simulink model "J52"  (R2015b)
settings: Solver=VariableStepAuto  StartTime=-10  StopTime=10.0  RelTol=1e-3
libraries: simulink x1
settings Model: Creator=Pouya  LastModifiedBy=Pouya

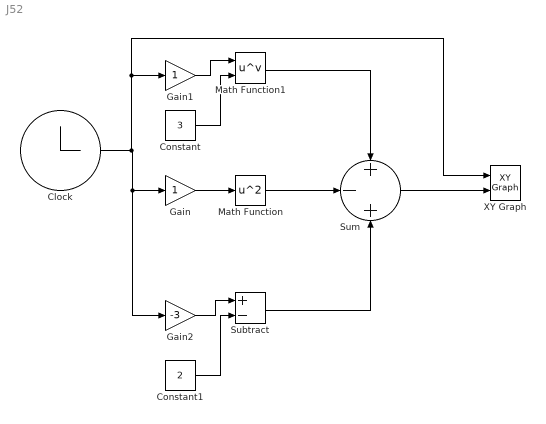
== system J52 ==
  Clock : Clock
  Constant : Constant  Value=3
  Constant1 : Constant  Value=2
  Gain : Gain
  Gain1 : Gain
  Gain2 : Gain  Gain=-3
  Math Function : Math  Operator=square  SaturateOnIntegerOverflow=on
  Math Function1 : Math  Operator=pow  SaturateOnIntegerOverflow=on
  Subtract : Sum  Inputs=+-
  Sum : Sum  Inputs=+-+
  XY Graph : simulink/Sinks/XY Graph  xmin=-4  xmax=4  ymin=-100  ymax=100  st=-1
  wires:
  Gain1/1 -> Math Function1/1
  Constant/1 -> Math Function1/2
  Gain/1 -> Math Function/1
  Clock/1 -> XY Graph/1, Gain1/1, Gain2/1, Gain/1
  Math Function1/1 -> Sum/1
  Math Function/1 -> Sum/2
  Gain2/1 -> Subtract/1
  Constant1/1 -> Subtract/2
  Sum/1 -> XY Graph/2
  Subtract/1 -> Sum/3
